simulink model "c281x_asyncscheduling_ert"  (R2021b)
settings: Solver=FixedStepDiscrete  StartTime=0.0  StopTime=inf  RelTol=1e-3  EnableMultiTasking=on
undefined symbols (not defined in the file or in its folder): Asymmetric, Up
libraries: c281xlib x4, simulink x4, c280xlib x2, demo_controls x1, c2000lib x1
settings Model: Creator=The MathWorks, Inc.  LastModifiedBy=The MathWorks, Inc.
settings SolverCC: AlgebraicLoopSolver=TrustRegion
settings DataIOCC: LimitDataPoints=on  SaveFormat=Array  SaveOutput=off  SaveTime=off  ReturnWorkspaceOutputs=off
settings OptimizationCC: ExpressionDepthLimit=2147483647  InitFltsAndDblsToZero=on  LifeSpan=inf  MaxStackSize=64  EfficientTunableParamExpr=on
settings DebuggingCC: UnderspecifiedInitializationDetection=Classic  MergeDetectMultiDrivingBlocksExec=none  SignalResolutionControl=TryResolveAllWithWarning  InheritedTsInSrcMsg=none  MultiTaskDSMMsg=warning  MultiTaskCondExecSysMsg=none  SigSpecEnsureSampleTimeMsg=none  IntegerOverflowMsg=none  FcnCallInpInsideContextMsg=warning  AllowSymbolicDim=off  StateNameClashWarn=warning  SFUnexpectedBacktrackingDiag=warning  SFNoUnconditionalDefaultTransitionDiag=warning  SFExecutionAtInitializationDiag=none  SFMachineParentedDataDiag=warning  IntegerSaturationMsg=none  ArithmeticOperatorsInVariantConditions=warning
settings HardwareCC: ProdBitPerChar=16  ProdBitPerInt=16  ProdBitPerPointer=32  ProdBitPerSizeT=32  ProdBitPerPtrDiffT=32  ProdLargestAtomicInteger=Integer  ProdLargestAtomicFloat=None  ProdWordSize=16  ProdHWDeviceType=Texas Instruments->C2000  TargetBitPerChar=16  TargetBitPerInt=16  TargetBitPerPointer=16  TargetLargestAtomicInteger=Integer  TargetIntDivRoundTo=Zero  TargetEndianess=LittleEndian  TargetWordSize=16  TargetHWDeviceType=Texas Instruments->C2000  ProdEqTarget=off
settings ModelReferenceCC: PropagateSignalLabelsOutOfModel=off
settings SFSimCC: SimUseLocalCustomCode=off  MATLABDynamicMemAlloc=off  CustomCodeUndefinedFunction=UseInterfaceOnly
settings RTWCC: Description=Embedded Coder  SystemTargetFile=ert.tlc  HardwareBoard=TI F281x  TemplateMakefile=ert_default_tmf  PostCodeGenCommand=; codertarget.postCodeGenHookCommand(h)  RTWUseLocalCustomCode=off  Toolchain=Texas Instruments Code Composer Studio (C2000)
settings CodeAppCC: IgnoreCustomStorageClasses=off  MaxIdLength=51  CustomSymbolStrType=$N$R$M  StateflowObjectComments=on  InternalIdentifier=Classic
settings ERTTargetCC: TargetFcnLib=ansi_tfl_tmw_new.mat  MultiwordLength=2048  ParMdlRefBuildCompliant=off  CompOptLevelCompliant=off  ConcurrentExecutionCompliant=off  CPPClassGenCompliant=off  ExtModeStaticAllocSize=2048  ExtModeMexFile=TIC2000ExternalModeOpen  ExtModeIntrfLevel=Level2 - Open  ConvertIfToSwitch=off  SuppressUnreachableDefaultCases=off
settings ConfigComp: CovMetricSettings=dw  CovSaveCumulativeToWorkspaceVar=on  CovSaveSingleToWorkspaceVar=on  CovExternalEMLEnable=off  CovSFcnEnable=off

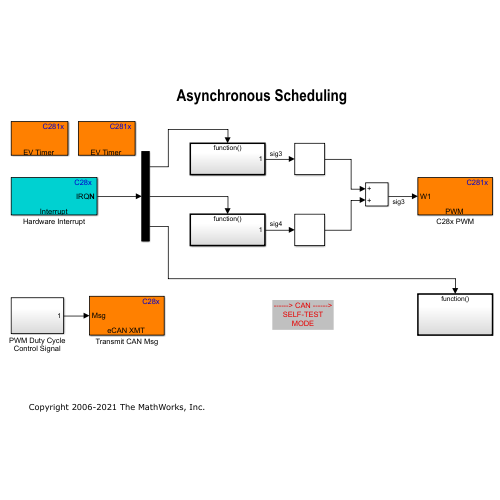
[thumbnail: Simulink's stored preview of the top-level diagram]
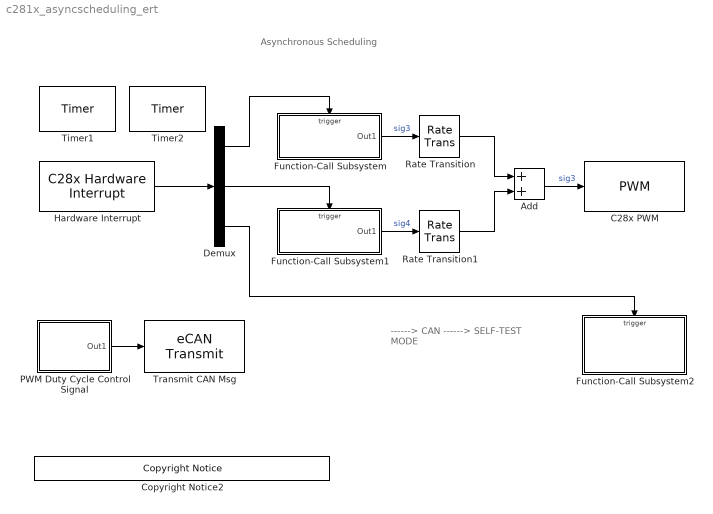
== system c281x_asyncscheduling_ert ==
  note: ------> CAN ------>
      | SELF-TEST
      | MODE
  note: Asynchronous Scheduling
  Add : Sum  SampleTime=0.001
  C28x PWM : c281xlib/PWM  useModule=B  timerSource=Specify via dialog  timerPeriod=32768  waveformType=Asymmetric(Up)  periodUnits=Clock cycles  preScaler=1/128  unit1Status=on  unit1Source=Input port  unit1Value=18500  unit2Status=off  unit2Source=Specify via dialog  unit2Value=18500  unit3Status=off  unit3Source=Specify via dialog  unit3Value=18500  dutyCycleUnits=Clock cycles  logicSource=Specify via dialog  unit1_1Logic=Active low  unit1_2Logic=Active high  unit2_1Logic=Active high  unit2_2Logic=Active low  unit3_1Logic=Active high  unit3_2Logic=Active low  enableDeadband1=off  enableDeadband2=off  enableDeadband3=off  deadbandPrescaler=1  deadbandPeriodSource=Specify via dialog  deadbandPeriod=1  adcStartTrigger=None  adcstartEvent=None
      settings: SourceProductBaseCode=TIC2000
  Copyright Notice2 : demo_controls/Copyright Notice  year=2006  prod=tic2000
      settings: SourceProductBaseCode=ME
  Demux : Demux  Outputs=3
  Function-Call Subsystem : Subsystem  TreatAsAtomicUnit=on
  Function-Call Subsystem1 : Subsystem  TreatAsAtomicUnit=on
  Function-Call Subsystem2 : Subsystem  TreatAsAtomicUnit=on
  Hardware Interrupt : c2000lib/Scheduling/C28x Hardware Interrupt  irqnumbers=[3 5 9]  pienumbers=[1 1 5]  irqpriorities=[50 60 30]  irqpreempts=[1]  showinput=off  dspchiptype=C281X
      settings: SourceProductBaseCode=TIC2000
  PWM Duty Cycle Control Signal : Subsystem
  Rate Transition : RateTransition  Deterministic=off
  Rate Transition1 : RateTransition  Deterministic=off
  Timer1 : c281xlib/Timer  module=B  timerAno=Timer 1  timerBno=Timer 4  clockSource=Internal  periodSource=Specify via dialog  period=20000  compareSource=Specify via dialog  compareValue=5000  countingMode=Up  preScaler=1/128  postPeriodInterrupt=on  postUnderflowInterrupt=off  postOverflowInterrupt=off  postCompareInterrupt=off
      settings: SourceProductBaseCode=TIC2000
  Timer2 : c281xlib/Timer  module=A  timerAno=Timer 2  timerBno=Timer 3  clockSource=Internal  periodSource=Specify via dialog  period=10000  compareSource=Specify via dialog  compareValue=5000  countingMode=Up  preScaler=1/128  postPeriodInterrupt=on  postUnderflowInterrupt=off  postOverflowInterrupt=off  postCompareInterrupt=off
      settings: SourceProductBaseCode=TIC2000
  Transmit CAN Msg : c280xlib/eCAN Transmit  chipFamily=C280x  useModule=eCAN_A  mailboxNo=5  messageID=bin2dec('111000111')  messageType=Standard (11-bit identifier)  enableBlockingMode=on  postInterrupt=off  interruptLine=0
      settings: SourceProductBaseCode=TIC2000
  wires:
  Function-Call Subsystem1/1(Out1) -> Rate Transition1/1  "sig4"
  Function-Call Subsystem/1(Out1) -> Rate Transition/1  "sig3"
  Demux/2 -> Function-Call Subsystem1/Trigger
  Rate Transition/1 -> Add/1
  Rate Transition1/1 -> Add/2
  Add/1 -> C28x PWM/1  "sig3"
  Demux/3 -> Function-Call Subsystem2/Trigger
  PWM Duty Cycle Control Signal/1(Out1) -> Transmit CAN Msg/1
  Hardware Interrupt/1 -> Demux/1
  Demux/1 -> Function-Call Subsystem/Trigger

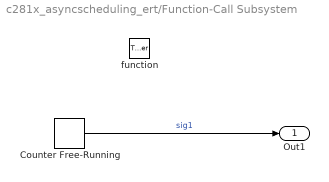
== system c281x_asyncscheduling_ert/Function-Call Subsystem ==
  function : TriggerPort  TriggerType=function-call  VariantControl=Variant
  Counter Free-Running : simulink/Sources/Counter Free-Running  NumBits=14  tsamp=-1
  Out1 : Outport  InitialOutput=0
  wires:
  Counter Free-Running/1 -> Out1/1  "sig1"

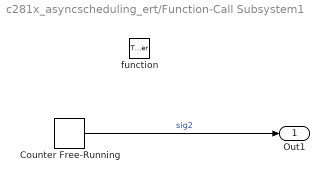
== system c281x_asyncscheduling_ert/Function-Call Subsystem1 ==
  function : TriggerPort  TriggerType=function-call  VariantControl=Variant
  Counter Free-Running : simulink/Sources/Counter Free-Running  NumBits=14  tsamp=-1
  Out1 : Outport  InitialOutput=0
  wires:
  Counter Free-Running/1 -> Out1/1  "sig2"

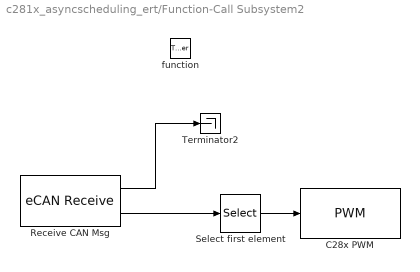
== system c281x_asyncscheduling_ert/Function-Call Subsystem2 ==
  function : TriggerPort  TriggerType=function-call  VariantControl=Variant
  C28x PWM : c281xlib/PWM  useModule=A  timerSource=Specify via dialog  timerPeriod=8000  waveformType=Asymmetric(Up)  periodUnits=Clock cycles  preScaler=1/128  unit1Status=on  unit1Source=Input port  unit1Value=18500  unit2Status=off  unit2Source=Specify via dialog  unit2Value=18500  unit3Status=off  unit3Source=Specify via dialog  unit3Value=18500  dutyCycleUnits=Clock cycles  logicSource=Specify via dialog  unit1_1Logic=Active low  unit1_2Logic=Active high  unit2_1Logic=Active high  unit2_2Logic=Active low  unit3_1Logic=Active high  unit3_2Logic=Active low  enableDeadband1=off  enableDeadband2=off  enableDeadband3=off  deadbandPrescaler=1  deadbandPeriodSource=Specify via dialog  deadbandPeriod=1  adcStartTrigger=None  adcstartEvent=None
      settings: SourceProductBaseCode=TIC2000
  Receive CAN Msg : c280xlib/eCAN Receive  chipFamily=C280x  useModule=eCAN_A  mailboxNo=0  messageID=bin2dec('111000111')  messageType=Standard (11-bit identifier)  enableAcceptanceFiltering=off  messageIDMask=0  sampleTime=-1  dataType=uint16  outputAction=Output last received values  initValue=0  outputMessageID=off  outputMessageLength=off  outputMessageTimeStamp=off  postInterrupt=on  interruptLine=0
      settings: SourceProductBaseCode=TIC2000
  Select first element : Selector  InputPortWidth=4  IndexOptions=Index vector (dialog)  Indices=[1]  OutputSizes=1
  Terminator2 : Terminator
  wires:
  Receive CAN Msg/2 -> Select first element/1
  Receive CAN Msg/1 -> Terminator2/1
  Select first element/1 -> C28x PWM/1

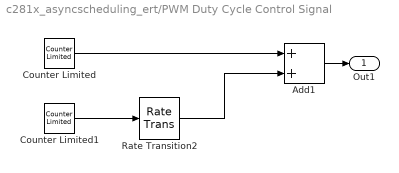
== system c281x_asyncscheduling_ert/PWM Duty Cycle Control Signal ==
  Add1 : Sum  OutDataTypeStr=Inherit: Inherit via back propagation
  Counter Limited : simulink/Sources/Counter Limited  uplimit=6000  tsamp=0.001
  Counter Limited1 : simulink/Sources/Counter Limited  uplimit=2000  tsamp=0.01
  Rate Transition2 : RateTransition  Deterministic=off
  Out1 : Outport
  wires:
  Counter Limited/1 -> Add1/1
  Counter Limited1/1 -> Rate Transition2/1
  Rate Transition2/1 -> Add1/2
  Add1/1 -> Out1/1
